simulink model "Homework_One_Question_One"  (R2020b)
settings: Solver=VariableStepAuto  StartTime=0.0  StopTime=2000.0  RelTol=1e-3
settings Model: Creator=jrsco  LastModifiedBy=jrsco

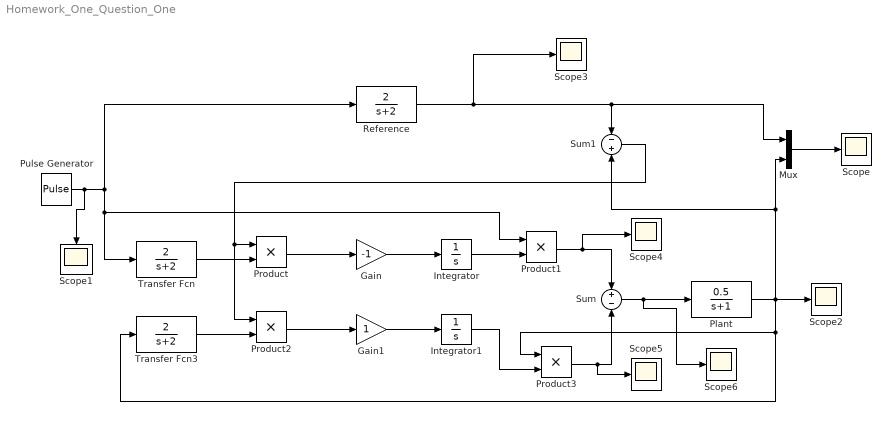
== system Homework_One_Question_One ==
  Gain : Gain  Gain=-1
  Gain1 : Gain
  Integrator : Integrator
  Integrator1 : Integrator
  Mux : Mux  Inputs=2
  Plant : TransferFcn  Numerator=[0.5]  Denominator=[1 1]
  Product{,1..3} (4 alike) : Product
  Pulse Generator : DiscretePulseGenerator  PulseType=Time based  Period=20  PulseWidth=50
  Reference : TransferFcn  Numerator=[2]  Denominator=[1 2]
  Scope{,1..6} (7 alike) : Scope
  Sum : Sum  Inputs=+-
  Sum1 : Sum  Inputs=-+
  Transfer Fcn : TransferFcn  Numerator=[2]  Denominator=[1 2]
  Transfer Fcn3 : TransferFcn  Numerator=[2]  Denominator=[1 2]
  wires:
  Pulse Generator/1 -> Scope1/1, Product1/1, Transfer Fcn/1, Reference/1
  Transfer Fcn/1 -> Product/2
  Product/1 -> Gain/1
  Gain/1 -> Integrator/1
  Integrator/1 -> Product1/2
  Product1/1 -> Scope4/1, Sum/1
  Product2/1 -> Gain1/1
  Gain1/1 -> Integrator1/1
  Integrator1/1 -> Product3/2
  Sum/1 -> Scope6/1, Plant/1
  Plant/1 -> Scope2/1, Mux/2, Sum1/2, Transfer Fcn3/1, Product3/1
  Product3/1 -> Scope5/1, Sum/2
  Reference/1 -> Scope3/1, Mux/1, Sum1/1
  Sum1/1 -> Product2/1, Product/1
  Mux/1 -> Scope/1
  Transfer Fcn3/1 -> Product2/2
